simulink model "Expt2_19EE3FP18_Swarnendu_QuesB_2020b"  (R2020b)
settings: Solver=FixedStepAuto  StartTime=0.0  StopTime=0.1  FixedStep=1e-7  MaxStep=1e-7  MinStep=1e-7  RelTol=1e-3
libraries: powerlib x16
settings Model: Creator=swarn  LastModifiedBy=swarn

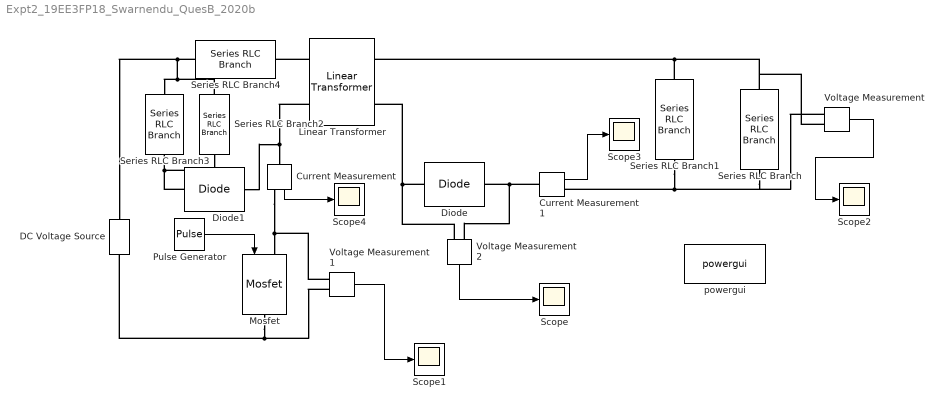
== system Expt2_19EE3FP18_Swarnendu_QuesB_2020b ==
  Current Measurement : powerlib/Measurements/Current Measurement  PhasorSimulation=off  OutputType=Complex  PSBequivalent=0
  Current Measurement1 : powerlib/Measurements/Current Measurement  PhasorSimulation=off  OutputType=Complex  PSBequivalent=0
  DC Voltage Source : powerlib/Electrical Sources/DC Voltage Source  Amplitude=24  Measurements=None
  Diode : powerlib/Power Electronics/Diode  Ron=1e-6  Lon=0  Vf=0  IC=0  UseSnubber=0  Rs=500  Cs=250e-9  Measurements=off
  Diode1 : powerlib/Power Electronics/Diode  Ron=1e-6  Lon=0  Vf=0  IC=0  UseSnubber=0  Rs=500  Cs=250e-9  Measurements=off
  Linear Transformer : powerlib/Elements/Linear Transformer  UNITS=SI  NominalPower=[ 200 1e5 ]  winding1=[24 0 0]  winding2=[9.6 0 0]  ThreeWindings=off  winding3=[3.15e+05 0.7938 0.084225]  RmLm=[1e12 20e-6]  Measurements=None  DataType=on
  Mosfet : powerlib/Power Electronics/Mosfet  Ron=1e-6  Lon=0  Rd=1e-6  Vfd=0  IC=0  Rs=1e5  Cs=inf  Measurements=off
  Pulse Generator : DiscretePulseGenerator  PulseType=Time based  Period=1e-5  PulseWidth=40
  Scope{,1..4} (5 alike) : Scope
  Series RLC Branch : powerlib/Elements/Series RLC Branch  LConnTagsString=__new0  RConnTagsString=__new0  BranchType=R  Resistance=1  Inductance=1e-3  SetiL0=off  InitialCurrent=0  Capacitance=1e-6  Setx0=off  InitialVoltage=0  Measurements=None
  Series RLC Branch1 : powerlib/Elements/Series RLC Branch  LConnTagsString=__new0  RConnTagsString=__new0  BranchType=C  Resistance=1  Inductance=1e-3  SetiL0=off  InitialCurrent=0  Capacitance=100e-6  Setx0=off  InitialVoltage=0  Measurements=None
  Series RLC Branch2 : powerlib/Elements/Series RLC Branch  LConnTagsString=__new0  RConnTagsString=__new0  BranchType=C  Resistance=3.5  Inductance=1e-3  SetiL0=off  InitialCurrent=0  Capacitance=50e-9  Setx0=off  InitialVoltage=0  Measurements=None
  Series RLC Branch3 : powerlib/Elements/Series RLC Branch  LConnTagsString=__new0  RConnTagsString=__new0  BranchType=R  Resistance=5e3  Inductance=1e-3  SetiL0=off  InitialCurrent=0  Capacitance=1e-6  Setx0=off  InitialVoltage=0  Measurements=None
  Series RLC Branch4 : powerlib/Elements/Series RLC Branch  LConnTagsString=__new0  RConnTagsString=__new0  BranchType=L  Resistance=3.5  Inductance=125e-9  SetiL0=off  InitialCurrent=0  Capacitance=1e-6  Setx0=off  InitialVoltage=0  Measurements=None
  Voltage Measurement : powerlib/Measurements/Voltage Measurement  PhasorSimulation=off  OutputType=Complex  PSBequivalent=0
  Voltage Measurement1 : powerlib/Measurements/Voltage Measurement  PhasorSimulation=off  OutputType=Complex  PSBequivalent=0
  Voltage Measurement2 : powerlib/Measurements/Voltage Measurement  PhasorSimulation=off  OutputType=Complex  PSBequivalent=0
  powergui : powerlib/powergui  Priority=1  SimulationMode=Discrete  SampleTime=1e-7  frequency=60  Iterations=50  frequencyindice=0  Pbase=100e6  ErrMax=1e-4  UnitsV=kV  UnitsW=MW  buscounter=0  FunctionMessages=off  echomessages=off  EnableUseOfTLC=off  CurrentSourceSwitches=off  DisableSnubberDevices=off  DisableRonSwitches=off  DisableVfSwitches=off  DisplayEquations=off  AutomaticDiscreteSolvers=off  SolverType=Tustin/Backward Euler (TBE)  Interpol=off  ExternalGateDelay=off  methode=off  Ts=100  x0status=blocks  SPID=on  SwTol=0  HookPort=off  NonlinearTolerance=1e-4  nMaxIteration=100  ContinueOnMaxIteration=off  RestoreLinks=warning  ResistiveCurrentMeasurement=off  Frange=[0:2:500]  Ylog=off  Xlog=on  ShowGrid=off  save=off  variable=ZData  structure=0  ZoomFFT=off  StartTime=0.0  cycles=1  DisplayStyle=1  fundamental=60  FreqAxis=off  MaxFrequency=1000  frequencyindicesteady=1  RmsSteady=1  display=off
  wires:
  Pulse Generator/1 -> Mosfet/1
  Voltage Measurement2/1 -> Scope/1
  Current Measurement1/1 -> Scope3/1
  Voltage Measurement1/1 -> Scope1/1
  Current Measurement/1 -> Scope4/1
  Voltage Measurement/1 -> Scope2/1
  connections:
  Mosfet/RConn1 -- Voltage Measurement1/LConn2 -- DC Voltage Source/LConn1
  Current Measurement/RConn1 -- Voltage Measurement1/LConn1 -- Mosfet/LConn1
  Linear Transformer/LConn2 -- Diode1/LConn1 -- Current Measurement/LConn1
  Series RLC Branch2/LConn1 -- DC Voltage Source/RConn1 -- Series RLC Branch4/LConn1 -- Series RLC Branch3/LConn1
  Current Measurement1/LConn1 -- Voltage Measurement2/LConn1 -- Diode/RConn1
  Diode/LConn1 -- Voltage Measurement2/LConn2 -- Linear Transformer/RConn2
  Series RLC Branch1/LConn1 -- Voltage Measurement/LConn2 -- Series RLC Branch/LConn1 -- Linear Transformer/RConn1
  Series RLC Branch1/RConn1 -- Voltage Measurement/LConn1 -- Series RLC Branch/RConn1 -- Current Measurement1/RConn1
  Diode1/RConn1 -- Series RLC Branch2/RConn1 -- Series RLC Branch3/RConn1
  Linear Transformer/LConn1 -- Series RLC Branch4/RConn1
